simulink model "test_RIP_R2019b"  (R2019b)
settings: Solver=FixedStepDiscrete  StartTime=0.0  StopTime=inf  FixedStep=0.001  RelTol=1e-3  EnableMultiTasking=on
values from neighbouring files (symbols this model uses):
  k = lqr(ss_model,Q,R)    [test_RIP.m]
libraries: simulink_extras x4, arduinolib x3, eeGeneralControl x2, arduinosensorlib x2, simulink x1
settings Model: SimulationMode=external  SILPILModeSetting=veronly  ExtModeTrigDuration=2  Creator=rob  LastModifiedBy=rob
settings OptimizationCC: EnhancedBackFolding=on  PassReuseOutputArgsAs=Individual arguments  ZeroExternalMemoryAtStartup=off  ZeroInternalMemoryAtStartup=off  MaxStackSize=64  OptimizeBlockOrder=speed  DifferentSizesBufferReuse=on  OptimizationCustomize=off  EfficientTunableParamExpr=on
settings DebuggingCC: ParameterTunabilityLossMsg=error  UnconnectedInputMsg=none  UnconnectedOutputMsg=none  UnconnectedLineMsg=none
settings HardwareCC: ProdBitPerPointer=32  ProdBitPerSizeT=32  ProdBitPerPtrDiffT=32  ProdLargestAtomicInteger=Long  ProdLargestAtomicFloat=Double  ProdWordSize=32  ProdHWDeviceType=ARM Compatible->ARM Cortex  UseEmbeddedCoderFeatures=off
settings ModelReferenceCC: EnableRefExpFcnMdlSchedulingChecks=off
settings SFSimCC: MATLABDynamicMemAlloc=off
settings RTWCC: SystemTargetFile=ert.tlc  HardwareBoard=ESP32-WROOM(Arduino Compatible)  TLCOptions="-aInlineSetEventsForThisBaseRateFcn=TLC_FALSE -aSuppressMultiTaskScheduler=TLC_FALSE  -aRateBasedStepFcn=0"  TemplateMakefile=ert_default_tmf  Toolchain=ESP32  BuildConfiguration=Faster Runs
settings CodeAppCC: ForceParamTrailComments=on  IgnoreCustomStorageClasses=off  OperatorAnnotations=on  SimulinkDataObjDesc=on  SFDataObjDesc=on  InsertBlockDesc=on
settings ERTTargetCC: SupportContinuousTime=on  SupportNonInlinedSFcns=on  SupportVariableSizeSignals=on  ExtModeTransport=3  ExtModeStaticAlloc=on  ExtModeStaticAllocSize=65536  ExtModeMexFile=ext_xcp  ExtModeIntrfLevel=Level2 - Open
settings SettingsController: UseSoCProfilerForTargets=0

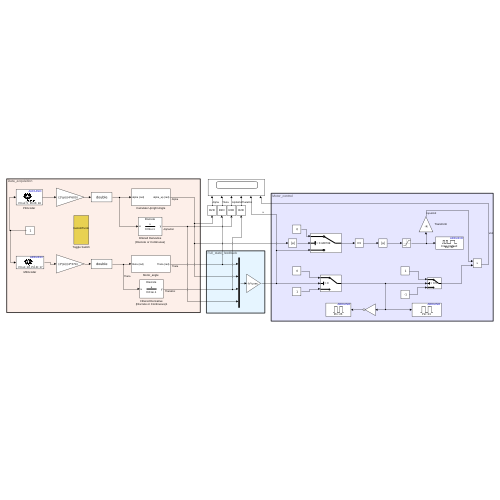
[thumbnail: Simulink's stored preview of the top-level diagram]
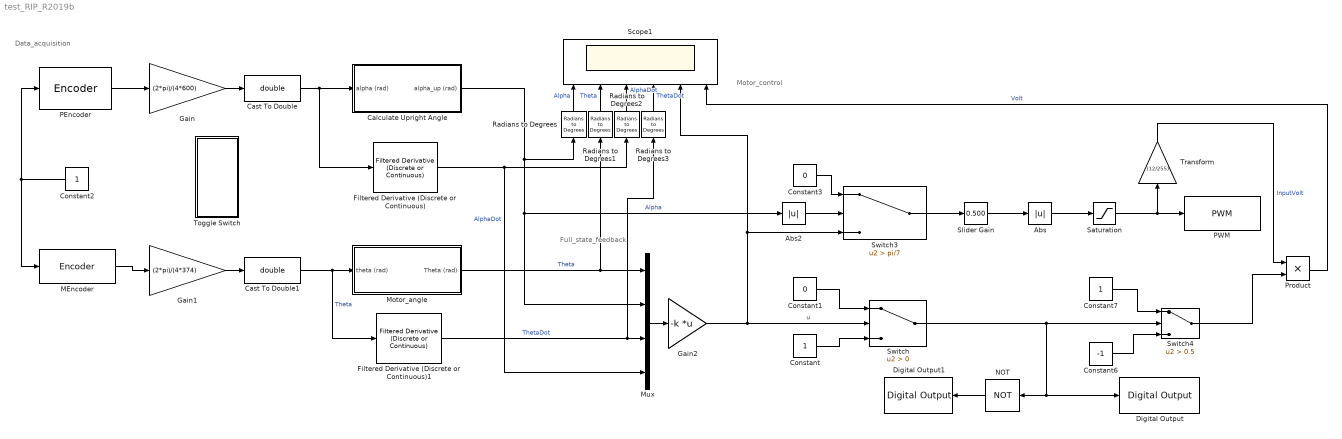
== system test_RIP_R2019b ==
  note: Full_state_feedback
  note: Data_acquisition
  note: Motor_control
  Abs : Abs
  Abs2 : Abs
  Calculate Upright Angle : Subsystem
  Cast To Double : DataTypeConversion  OutDataTypeStr=double
  Cast To Double1 : DataTypeConversion  OutDataTypeStr=double
  Constant : Constant
  Constant1 : Constant  Value=0
  Constant2 : Constant
  Constant3 : Constant  Value=0
  Constant6 : Constant  Value=-1
  Constant7 : Constant
  Digital Output : arduinolib/Digital Output  pinNumber=33  Direction=output  blockPlatform=arduino
  Digital Output1 : arduinolib/Digital Output  pinNumber=25  Direction=output  blockPlatform=arduino
  Filtered Derivative (Discrete or Continuous) : eeGeneralControl/Filtered Derivative (Discrete or Continuous)  K=1  T=0.01  B=inf  A=-inf  minRatio=10  init_option=Inherited from block input  x0=0  Ts=-1
  Filtered Derivative (Discrete or Continuous)1 : eeGeneralControl/Filtered Derivative (Discrete or Continuous)  K=1  T=0.01  B=inf  A=-inf  minRatio=10  init_option=Inherited from block input  x0=0  Ts=-1
  Gain : Gain  Gain=(2*pi)/(4*600)
  Gain1 : Gain  Gain=(2*pi)/(4*374)
  Gain2 : Gain  Gain=-k  Multiplication=Matrix(K*u) (u vector)
  MEncoder : arduinosensorlib/Encoder  InputA=16  InputB=17  Mode=Reset by external signal  SampleTime=-1
  Motor_angle : Subsystem
  Mux : Mux
  NOT : Logic  Operator=NOT  IconShape=distinctive  AllPortsSameDT=off  OutDataTypeStr=boolean
  PEncoder : arduinosensorlib/Encoder  InputA=5  InputB=18  Mode=Reset by external signal  SampleTime=-1
  PWM : arduinolib/PWM  pinNumber=32  frequencyType=Default  desiredFrequency=490.2  achievableFrequency=490.2
  Product : Product
  Radians to Degrees{,1..3} (4 alike) : simulink_extras/Transformations/Radians to Degrees
  Saturation : Saturate  UpperLimit=255  LowerLimit=0
  Scope1 : Scope  NumInputPorts=6
  Slider Gain : simulink/Math Operations/Slider Gain  gain=0.500  low=0.5  high=1.5
  Switch : Switch  Criteria=u2 > Threshold
  Switch3 : Switch  Criteria=u2 > Threshold  Threshold=pi/7
  Switch4 : Switch  Criteria=u2 > Threshold  Threshold=0.5
  Toggle Switch : Subsystem  Description=Replaced Block  mask(Replaced Block){}
      mask help: This block has been replaced with an empty subsystem because it used functionality that is unavailable in Simulink R2019b.
      mask Display: fprintf('Replaced: %s\n','CustomTuningWebBlock')
  Transform : Gain  Gain=(12/255)
  wires:
  PEncoder/1 -> Gain/1
  Gain1/1 -> Cast To Double1/1
  Slider Gain/1 -> Abs/1
  Constant1/1 -> Switch/1
  Gain2/1 -> Switch/2, Switch3/3, Scope1/5  "u"
  Constant7/1 -> Switch4/1
  Switch/1 -> NOT/1, Digital Output/1, Switch4/2
  Cast To Double/1 -> Filtered Derivative (Discrete or Continuous)/1, Calculate Upright Angle/1(alpha (rad))
  Radians to Degrees3/1 -> Scope1/4  "ThetaDot"
  Abs/1 -> Saturation/1
  Mux/1 -> Gain2/1
  Transform/1 -> Product/1  "InputVolt"
  Switch4/1 -> Product/2
  Filtered Derivative (Discrete or Continuous)/1 -> Radians to Degrees2/1, Mux/4  "AlphaDot"
  Switch3/1 -> Slider Gain/1
  Calculate Upright Angle/1(alpha_up (rad)) -> Mux/2, Abs2/1, Radians to Degrees/1  "Alpha"
  Gain/1 -> Cast To Double/1
  Constant6/1 -> Switch4/3
  Saturation/1 -> PWM/1, Transform/1
  Radians to Degrees1/1 -> Scope1/2  "Theta"
  MEncoder/1 -> Gain1/1
  Radians to Degrees/1 -> Scope1/1  "Alpha"
  Abs2/1 -> Switch3/2
  Radians to Degrees2/1 -> Scope1/3  "AlphaDot"
  NOT/1 -> Digital Output1/1
  Constant3/1 -> Switch3/1
  Cast To Double1/1 -> Filtered Derivative (Discrete or Continuous)1/1, Motor_angle/1(theta (rad))  "Theta"
  Filtered Derivative (Discrete or Continuous)1/1 -> Mux/3, Radians to Degrees3/1  "ThetaDot"
  Constant/1 -> Switch/3
  Product/1 -> Scope1/6  "Volt"
  Motor_angle/1(Theta (rad)) -> Mux/1, Radians to Degrees1/1  "Theta"
  Constant2/1 -> PEncoder/1, MEncoder/1

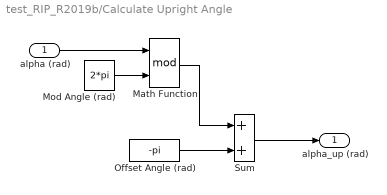
== system test_RIP_R2019b/Calculate Upright Angle ==
  alpha (rad) : Inport
  Math Function : Math  Operator=mod  SignedPower=on  SaturateOnIntegerOverflow=on
  Mod Angle (rad) : Constant  Value=2*pi
  Offset Angle (rad) : Constant  Value=-pi
  Sum : Sum  InputSameDT=on  SaturateOnIntegerOverflow=on  OutDataTypeStr=Inherit: Same as first input
  alpha_up (rad) : Outport  VectorParamsAs1DForOutWhenUnconnected=off
  wires:
  Math Function/1 -> Sum/1
  alpha (rad)/1 -> Math Function/1
  Offset Angle (rad)/1 -> Sum/2
  Mod Angle (rad)/1 -> Math Function/2
  Sum/1 -> alpha_up (rad)/1

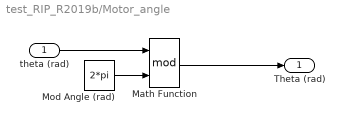
== system test_RIP_R2019b/Motor_angle ==
  theta (rad) : Inport
  Math Function : Math  Operator=mod  SignedPower=on  SaturateOnIntegerOverflow=on
  Mod Angle (rad) : Constant  Value=2*pi
  Theta (rad) : Outport  VectorParamsAs1DForOutWhenUnconnected=off
  wires:
  Mod Angle (rad)/1 -> Math Function/2
  theta (rad)/1 -> Math Function/1
  Math Function/1 -> Theta (rad)/1

== system test_RIP_R2019b/Toggle Switch ==
